simulink model "AM_signal2019a"  (R2019a)
settings: Solver=VariableStepAuto  StartTime=0.0  StopTime=10.0  RelTol=1e-3
libraries: commchan3 x1, dsparch4 x1, commanapbnd3 x1
settings Model: Creator=Kai  LastModifiedBy=Kai

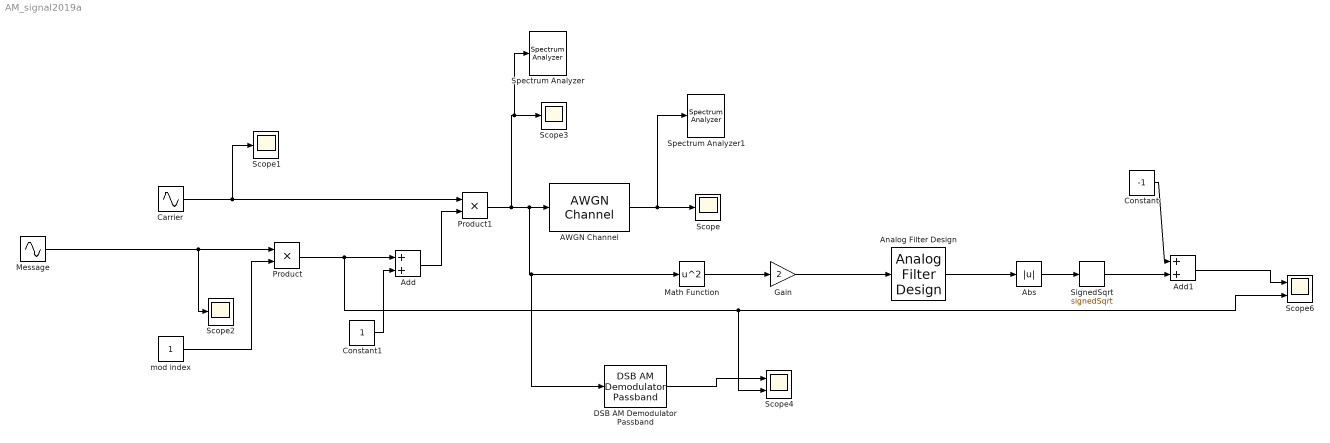
== system AM_signal2019a ==
  AWGN Channel : commchan3/AWGN Channel  InputProcessing=Columns as channels (frame based)  seed=67  noiseMode="Signal to noise ratio  (SNR)"  EbNodB=10  EsNodB=10  SNRdB=3  bitsPerSym=1  Ps=1  Tsym=1  variance=1
      settings: SourceProductName=Communications Toolbox
  Abs : Abs
  Add : Sum
  Add1 : Sum
  Analog Filter Design : dsparch4/Analog Filter Design  method=Butterworth  filttype=Lowpass  N=8  Wlo=2*pi*10  Whi=80  Rp=2  Rs=40
  Carrier : Sin  Frequency=2*pi*10  SampleTime=1/5000
  Constant : Constant  Value=-1
  Constant1 : Constant
  DSB AM Demodulator Passband : commanapbnd3/DSB AM Demodulator Passband  Fc=62.8  Ph=0  method=Butterworth  n=4  cf=62.8  Rp=0.1  Rs=50  Offset=1
      settings: SourceProductName=Communications Toolbox  SourceProductBaseCode=CM
  Gain : Gain  Gain=2
  Math Function : Math  Operator=square  SaturateOnIntegerOverflow=on
  "Message " : Sin  Frequency=2*pi  SampleTime=1/5000
  Product : Product
  Product1 : Product
  Scope{,1..3} (4 alike) : Scope
  Scope4 : Scope  NumInputPorts=2
  Scope6 : Scope  NumInputPorts=2
  SignedSqrt : Sqrt  Operator=signedSqrt  IntermediateResultsDataTypeStr=single  SaturateOnIntegerOverflow=on
  Spectrum Analyzer : SpectrumAnalyzer
  Spectrum Analyzer1 : SpectrumAnalyzer
  mod index : Constant
  wires:
  "Message "/1 -> Scope2/1, Product/1
  mod index/1 -> Product/2
  Carrier/1 -> Product1/1, Scope1/1
  Product/1 -> Scope4/2, Scope6/2, Add/1
  Constant1/1 -> Add/2
  Add/1 -> Product1/2
  AWGN Channel/1 -> Spectrum Analyzer1/1, Scope/1
  Product1/1 -> Spectrum Analyzer/1, Scope3/1, DSB AM Demodulator Passband/1, Math Function/1, AWGN Channel/1
  Analog Filter Design/1 -> Abs/1
  Abs/1 -> SignedSqrt/1
  Math Function/1 -> Gain/1
  Gain/1 -> Analog Filter Design/1
  SignedSqrt/1 -> Add1/2
  Constant/1 -> Add1/1
  Add1/1 -> Scope6/1
  DSB AM Demodulator Passband/1 -> Scope4/1
